simulink library "xrbsComm_r4"  (Simulink 7.1)
PreLoadFcn:
  | warning('off','MATLAB:mex:deprecatedExtension');xlmeta;com.xilinx.sysgen.util.StrategyUtil.loadAllStrategyNames();
undefined symbols (not defined in the file or in its folder): calc_path_data, gcbh, mfcm_matrix_rom, oct2dec, xlBlockLoadCallback
libraries: xbsIndex_r4 x851, mfcm_block_lib_v1 x5, xrbsComm_r4 x1, mfcm_misc_lib_v1 x1
(part 3 of 8)

== system xrbsComm_r4/White Gaussian  Noise Generator/Box-Muller1/f/lfsr_29_2 ==
  note: 4-Bit Leap-Forward LFSR G(X) = X^29 + X^2 + 1
  reset : Inport  OutDataType=sfix(16)  OutScaling=2^0
  Concat : xbsIndex_r4/Concat  num_inputs=2  dbl_ovrd=off  block_type=concat
      settings: block_version=VER_STRING_GOES_HERE
  Concat1 : xbsIndex_r4/Concat  num_inputs=2  dbl_ovrd=off  block_type=concat
      settings: block_version=VER_STRING_GOES_HERE
  Concat2 : xbsIndex_r4/Concat  num_inputs=2  dbl_ovrd=off  block_type=concat
      settings: block_version=VER_STRING_GOES_HERE
  Logical{,1..3} (4 alike) : xbsIndex_r4/Logical  logical_function=XOR  inputs=2  en=off  latency=0  precision=User Defined  arith_type=Unsigned  n_bits=1  bin_pt=0  align_bp=on  dbl_ovrd=off  block_type=logical
      settings: xl_area=[0, 0, 0, 0, 0, 0, 0]  block_version=VER_STRING_GOES_HERE
  x : xbsIndex_r4/Register  init=init(1)  rst=on  en=off  dbl_ovrd=off  block_type=register
      settings: xl_area=[0, 0, 0, 0, 0, 0, 0]  block_version=VER_STRING_GOES_HERE
  x2 : xbsIndex_r4/Register  init=init(2)  rst=on  en=off  dbl_ovrd=off  block_type=register
      settings: xl_area=[0, 0, 0, 0, 0, 0, 0]  block_version=VER_STRING_GOES_HERE
  x3 : xbsIndex_r4/Register  init=init(3)  rst=on  en=off  dbl_ovrd=off  block_type=register
      settings: xl_area=[0, 0, 0, 0, 0, 0, 0]  block_version=VER_STRING_GOES_HERE
  x4 : xbsIndex_r4/Register  init=init(4)  rst=on  en=off  dbl_ovrd=off  block_type=register
      settings: xl_area=[0, 0, 0, 0, 0, 0, 0]  block_version=VER_STRING_GOES_HERE
  x5 : Subsystem  mask{init=init(5:4:29)}
  x6 : Subsystem  mask{init=init(6:4:26)}
  x7 : Subsystem  mask{init=init(7:4:27)}
  x8 : Subsystem  mask{init=init(8:4:28)}
  " " : Outport  OutDataType=sfix(16)  OutScaling=2^0
  wires:
  Logical/1 -> x5/1(" ")
  Logical1/1 -> x6/1(" ")
  Logical2/1 -> x7/1(" ")
  Logical3/1 -> x8/1(" ")
  x5/1(z-7) -> x/1, Logical3/2
  x6/1(z-6) -> x2/1, Logical/2
  x7/1(z-6) -> x3/1
  x8/1(z-6) -> x4/1
  x/1 -> Logical1/1, Concat/1
  x2/1 -> Concat/2, Logical2/1
  Concat/1 -> Concat2/1
  x3/1 -> Concat1/1, Logical3/1, Logical1/2
  x4/1 -> Concat1/2, Logical2/2, Logical/1
  Concat1/1 -> Concat2/2
  Concat2/1 -> " "/1
  reset/1 -> x8/2(reset), x7/2(reset), x6/2(reset), x5/2(reset), x/2, x2/2, x3/2, x4/2

== system xrbsComm_r4/White Gaussian  Noise Generator/Box-Muller1/f/lfsr_31_2 ==
  note: 4-Bit Leap-Forward LFSR G(X) = X^31 + X^3 + 1
  reset : Inport  OutDataType=sfix(16)  OutScaling=2^0
  Concat : xbsIndex_r4/Concat  num_inputs=2  dbl_ovrd=off  block_type=concat
      settings: block_version=VER_STRING_GOES_HERE
  Concat1 : xbsIndex_r4/Concat  num_inputs=2  dbl_ovrd=off  block_type=concat
      settings: block_version=VER_STRING_GOES_HERE
  Concat2 : xbsIndex_r4/Concat  num_inputs=2  dbl_ovrd=off  block_type=concat
      settings: block_version=VER_STRING_GOES_HERE
  Logical{,1..3} (4 alike) : xbsIndex_r4/Logical  logical_function=XOR  inputs=2  en=off  latency=0  precision=User Defined  arith_type=Unsigned  n_bits=1  bin_pt=0  align_bp=on  dbl_ovrd=off  block_type=logical
      settings: xl_area=[0, 0, 0, 0, 0, 0, 0]  block_version=VER_STRING_GOES_HERE
  x : xbsIndex_r4/Register  init=init(1)  rst=on  en=off  dbl_ovrd=off  block_type=register
      settings: xl_area=[0, 0, 0, 0, 0, 0, 0]  block_version=VER_STRING_GOES_HERE
  x2 : xbsIndex_r4/Register  init=init(2)  rst=on  en=off  dbl_ovrd=off  block_type=register
      settings: xl_area=[0, 0, 0, 0, 0, 0, 0]  block_version=VER_STRING_GOES_HERE
  x3 : xbsIndex_r4/Register  init=init(3)  rst=on  en=off  dbl_ovrd=off  block_type=register
      settings: xl_area=[0, 0, 0, 0, 0, 0, 0]  block_version=VER_STRING_GOES_HERE
  x4 : xbsIndex_r4/Register  init=init(4)  rst=on  en=off  dbl_ovrd=off  block_type=register
      settings: xl_area=[0, 0, 0, 0, 0, 0, 0]  block_version=VER_STRING_GOES_HERE
  x5 : Subsystem  mask{init=init(5:4:29)}
  x6 : Subsystem  mask{init=init(6:4:30)}
  x7 : Subsystem  mask{init=init(7:4:31)}
  x8 : Subsystem  mask{init=init(8:4:28)}
  " " : Outport  OutDataType=sfix(16)  OutScaling=2^0
  wires:
  Logical/1 -> x5/1(" ")
  Logical1/1 -> x6/1(" ")
  Logical2/1 -> x7/1(" ")
  Logical3/1 -> x8/1(" ")
  x5/1(z-7) -> Logical/1, x/1
  x6/1(z-7) -> Logical1/1, x2/1
  x7/1(z-7) -> x3/1, Logical2/1
  x8/1(z-6) -> x4/1
  x/1 -> Concat/1, Logical3/1
  x2/1 -> Concat/2, Logical/2
  Concat/1 -> Concat2/1
  x3/1 -> Concat1/1, Logical1/2
  x4/1 -> Logical2/2, Concat1/2, Logical3/2
  Concat1/1 -> Concat2/2
  Concat2/1 -> " "/1
  reset/1 -> x5/2(reset), x6/2(reset), x7/2(reset), x8/2(reset), x/2, x2/2, x3/2, x4/2

== system xrbsComm_r4/White Gaussian  Noise Generator/Box-Muller1/f/lfsr_41_2 ==
  note: 4-Bit Leap-Forward LFSR G(X) = X^41 + X^3 + 1
  reset : Inport  OutDataType=sfix(16)  OutScaling=2^0
  Concat : xbsIndex_r4/Concat  num_inputs=2  dbl_ovrd=off  block_type=concat
      settings: block_version=VER_STRING_GOES_HERE
  Concat1 : xbsIndex_r4/Concat  num_inputs=2  dbl_ovrd=off  block_type=concat
      settings: block_version=VER_STRING_GOES_HERE
  Concat2 : xbsIndex_r4/Concat  num_inputs=2  dbl_ovrd=off  block_type=concat
      settings: block_version=VER_STRING_GOES_HERE
  Logical{,1..3} (4 alike) : xbsIndex_r4/Logical  logical_function=XOR  inputs=2  en=off  latency=0  precision=User Defined  arith_type=Unsigned  n_bits=1  bin_pt=0  align_bp=on  dbl_ovrd=off  block_type=logical
      settings: xl_area=[0, 0, 0, 0, 0, 0, 0]  block_version=VER_STRING_GOES_HERE
  x : xbsIndex_r4/Register  init=init(1)  rst=on  en=off  dbl_ovrd=off  block_type=register
      settings: xl_area=[0, 0, 0, 0, 0, 0, 0]  block_version=VER_STRING_GOES_HERE
  x1 : Subsystem  mask{init=init(6:4:38)}
  x2 : xbsIndex_r4/Register  init=init(2)  rst=on  en=off  dbl_ovrd=off  block_type=register
      settings: xl_area=[0, 0, 0, 0, 0, 0, 0]  block_version=VER_STRING_GOES_HERE
  x3 : xbsIndex_r4/Register  init=init(3)  rst=on  en=off  dbl_ovrd=off  block_type=register
      settings: xl_area=[0, 0, 0, 0, 0, 0, 0]  block_version=VER_STRING_GOES_HERE
  x4 : xbsIndex_r4/Register  init=init(4)  rst=on  en=off  dbl_ovrd=off  block_type=register
      settings: xl_area=[0, 0, 0, 0, 0, 0, 0]  block_version=VER_STRING_GOES_HERE
  x5 : Subsystem  mask{init=init(5:4:41)}
  x6 : Subsystem  mask{init=init(7:4:39)}
  x7 : Subsystem  mask{init=init(8:4:40)}
  " " : Outport  OutDataType=sfix(16)  OutScaling=2^0
  wires:
  Logical/1 -> x5/1(" ")
  Logical1/1 -> x1/1(" ")
  Logical2/1 -> x6/1(" ")
  Logical3/1 -> x7/1(" ")
  x5/1(z-10) -> x/1, Logical2/2
  x1/1(z-9) -> x2/1, Logical3/2
  x6/1(z-9) -> x3/1, Logical/2
  x7/1(z-9) -> x4/1
  x/1 -> Logical1/1, Concat/1
  x2/1 -> Concat/2, Logical2/1
  Concat/1 -> Concat2/1
  x3/1 -> Concat1/1, Logical3/1
  x4/1 -> Concat1/2, Logical1/2, Logical/1
  Concat1/1 -> Concat2/2
  Concat2/1 -> " "/1
  reset/1 -> x5/2(reset), x1/2(reset), x6/2(reset), x7/2(reset), x/2, x2/2, x3/2, x4/2

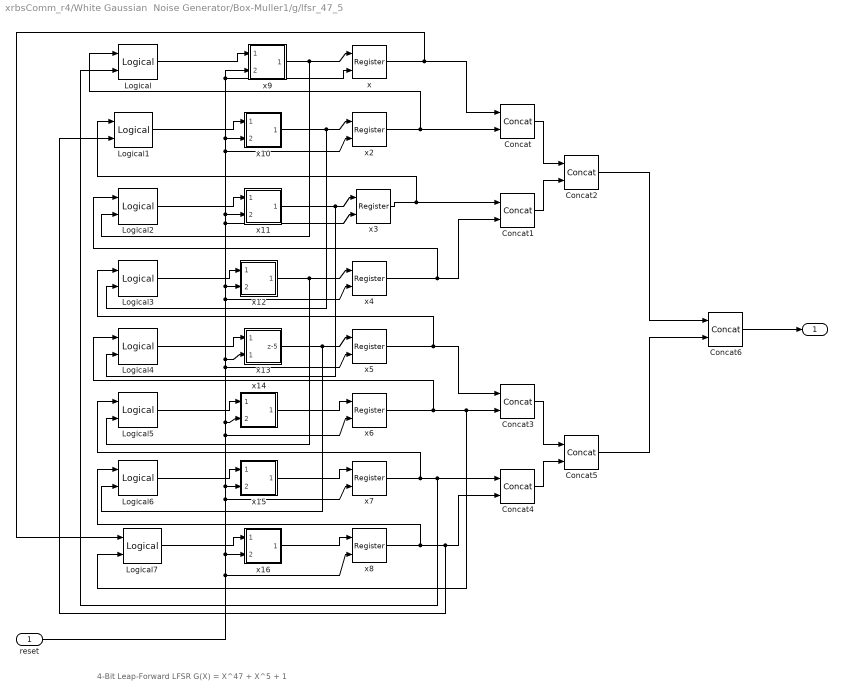
== system xrbsComm_r4/White Gaussian  Noise Generator/Box-Muller1/g/lfsr_47_5 ==
  note: 4-Bit Leap-Forward LFSR G(X) = X^47 + X^5 + 1
  reset : Inport  OutDataType=sfix(16)  OutScaling=2^0
  Concat{,1..6} (7 alike) : xbsIndex_r4/Concat  num_inputs=2  dbl_ovrd=off  block_type=concat
      settings: block_version=VER_STRING_GOES_HERE
  Logical{,1..7} (8 alike) : xbsIndex_r4/Logical  logical_function=XOR  inputs=2  en=off  latency=0  precision=User Defined  arith_type=Unsigned  n_bits=1  bin_pt=0  align_bp=on  dbl_ovrd=off  block_type=logical
      settings: xl_area=[0, 0, 0, 0, 0, 0, 0]  block_version=VER_STRING_GOES_HERE
  x : xbsIndex_r4/Register  init=init(1)  rst=on  en=off  dbl_ovrd=off  block_type=register
      settings: xl_area=[0, 0, 0, 0, 0, 0, 0]  block_version=VER_STRING_GOES_HERE
  x10 : Subsystem  mask{init=init(10:8:42)}
  x11 : Subsystem  mask{init=init(11:8:43)}
  x12 : Subsystem  mask{init=init(12:8:44)}
  x13 : Subsystem  mask{init=init(13:8:45)}
  x14 : Subsystem  mask{init=init(14:8:46)}
  x15 : Subsystem  mask{init=init(15:8:47)}
  x16 : Subsystem  mask{init=init(16:8:40)}
  x2 : xbsIndex_r4/Register  init=init(2)  rst=on  en=off  dbl_ovrd=off  block_type=register
      settings: xl_area=[0, 0, 0, 0, 0, 0, 0]  block_version=VER_STRING_GOES_HERE
  x3 : xbsIndex_r4/Register  init=init(3)  rst=on  en=off  dbl_ovrd=off  block_type=register
      settings: xl_area=[0, 0, 0, 0, 0, 0, 0]  block_version=VER_STRING_GOES_HERE
  x4 : xbsIndex_r4/Register  init=init(4)  rst=on  en=off  dbl_ovrd=off  block_type=register
      settings: xl_area=[0, 0, 0, 0, 0, 0, 0]  block_version=VER_STRING_GOES_HERE
  x5 : xbsIndex_r4/Register  init=init(5)  rst=on  en=off  dbl_ovrd=off  block_type=register
      settings: xl_area=[0, 0, 0, 0, 0, 0, 0]  block_version=VER_STRING_GOES_HERE
  x6 : xbsIndex_r4/Register  init=init(6)  rst=on  en=off  dbl_ovrd=off  block_type=register
      settings: xl_area=[0, 0, 0, 0, 0, 0, 0]  block_version=VER_STRING_GOES_HERE
  x7 : xbsIndex_r4/Register  init=init(7)  rst=on  en=off  dbl_ovrd=off  block_type=register
      settings: xl_area=[0, 0, 0, 0, 0, 0, 0]  block_version=VER_STRING_GOES_HERE
  x8 : xbsIndex_r4/Register  init=init(8)  rst=on  en=off  dbl_ovrd=off  block_type=register
      settings: xl_area=[0, 0, 0, 0, 0, 0, 0]  block_version=VER_STRING_GOES_HERE
  x9 : Subsystem  mask{init=init(9:8:41)}
  " " : Outport  OutDataType=sfix(16)  OutScaling=2^0
  wires:
  Logical/1 -> x9/1(" ")
  x9/1(z-5) -> x/1, Logical2/2
  x/1 -> Concat/1, Logical7/1
  x2/1 -> Concat/2, Logical/1
  Concat/1 -> Concat2/1
  x3/1 -> Concat1/1, Logical1/1
  x4/1 -> Concat1/2, Logical2/1
  Concat1/1 -> Concat2/2
  Logical1/1 -> x10/1("  ")
  x10/1(z-5) -> x2/1, Logical3/2
  Logical2/1 -> x11/1(" ")
  x11/1(z-5) -> x3/1, Logical4/2
  Logical3/1 -> x12/1(" ")
  x12/1(z-5) -> x4/1, Logical5/2
  Logical4/1 -> x13/1(" ")
  x13/1(z-5) -> x5/1, Logical6/2
  Logical5/1 -> x14/1(" ")
  x14/1(z-5) -> x6/1
  Logical6/1 -> x15/1(" ")
  x15/1(z-5) -> x7/1
  Logical7/1 -> x16/1(" ")
  x16/1(z-4) -> x8/1
  x6/1 -> Logical4/1, Concat3/2, Logical7/2
  Concat3/1 -> Concat5/1
  Concat4/1 -> Concat5/2
  x5/1 -> Concat3/1, Logical3/1
  x7/1 -> Concat4/1, Logical/2, Logical5/1
  x8/1 -> Concat4/2, Logical1/2, Logical6/1
  Concat2/1 -> Concat6/1
  Concat5/1 -> Concat6/2
  Concat6/1 -> " "/1
  reset/1 -> x9/2(reset), x/2, x10/2(reset), x2/2, x11/2(reset), x3/2, x12/2(reset), x4/2, x13/2(" 1"), x5/2, x14/2(reset), x6/2, x15/2(reset), x7/2, x16/2(reset), x8/2

== system xrbsComm_r4/White Gaussian  Noise Generator/Box-Muller2/fr1/iszero ==
  " " : Inport  OutDataType=sfix(16)  OutScaling=2^0
  "const " : xbsIndex_r4/Constant  arith_type=Unsigned  const=0  n_bits=4  bin_pt=0  explicit_period=off  period=1  equ=P=C  opselect=C  inp2=PCIN>>17  opr=+  inp1=P  carry=CIN  dbl_ovrd=off  block_type=constant
      settings: block_version=VER_STRING_GOES_HERE
  sel1 : xbsIndex_r4/Relational  mode=a=b  en=off  latency=1  dbl_ovrd=off  block_type=relational
      settings: xl_area=[0, 0, 0, 0, 0, 0, 0]  block_version=VER_STRING_GOES_HERE
  eq : Outport  OutDataType=sfix(16)  OutScaling=2^0
  wires:
  "const "/1 -> sel1/2
  " "/1 -> sel1/1
  sel1/1 -> eq/1

== system xrbsComm_r4/White Gaussian  Noise Generator/Box-Muller2/fr1/iszero1 ==
  " " : Inport  OutDataType=sfix(16)  OutScaling=2^0
  Constant1 : xbsIndex_r4/Constant  arith_type=Unsigned  const=0  n_bits=4  bin_pt=0  explicit_period=off  period=1  equ=P=C  opselect=C  inp2=PCIN>>17  opr=+  inp1=P  carry=CIN  dbl_ovrd=off  block_type=constant
      settings: block_version=VER_STRING_GOES_HERE
  sel2 : xbsIndex_r4/Relational  mode=a=b  en=off  latency=1  dbl_ovrd=off  block_type=relational
      settings: xl_area=[0, 0, 0, 0, 0, 0, 0]  block_version=VER_STRING_GOES_HERE
  eq : Outport  OutDataType=sfix(16)  OutScaling=2^0
  wires:
  Constant1/1 -> sel2/2
  " "/1 -> sel2/1
  sel2/1 -> eq/1

== system xrbsComm_r4/White Gaussian  Noise Generator/Box-Muller2/fr1/iszero2 ==
  " " : Inport  OutDataType=sfix(16)  OutScaling=2^0
  Constant3 : xbsIndex_r4/Constant  arith_type=Unsigned  const=0  n_bits=4  bin_pt=0  explicit_period=off  period=1  equ=P=C  opselect=C  inp2=PCIN>>17  opr=+  inp1=P  carry=CIN  dbl_ovrd=off  block_type=constant
      settings: block_version=VER_STRING_GOES_HERE
  sel3 : xbsIndex_r4/Relational  mode=a=b  en=off  latency=1  dbl_ovrd=off  block_type=relational
      settings: xl_area=[0, 0, 0, 0, 0, 0, 0]  block_version=VER_STRING_GOES_HERE
  eq : Outport  OutDataType=sfix(16)  OutScaling=2^0
  wires:
  Constant3/1 -> sel3/2
  " "/1 -> sel3/1
  sel3/1 -> eq/1

== system xrbsComm_r4/White Gaussian  Noise Generator/Box-Muller2/fr1/iszero3 ==
  " " : Inport  OutDataType=sfix(16)  OutScaling=2^0
  Constant : xbsIndex_r4/Constant  arith_type=Unsigned  const=0  n_bits=4  bin_pt=0  explicit_period=off  period=1  equ=P=C  opselect=C  inp2=PCIN>>17  opr=+  inp1=P  carry=CIN  dbl_ovrd=off  block_type=constant
      settings: block_version=VER_STRING_GOES_HERE
  sel4 : xbsIndex_r4/Relational  mode=a=b  en=off  latency=1  dbl_ovrd=off  block_type=relational
      settings: xl_area=[0, 0, 0, 0, 0, 0, 0]  block_version=VER_STRING_GOES_HERE
  eq : Outport  OutDataType=sfix(16)  OutScaling=2^0
  wires:
  Constant/1 -> sel4/2
  " "/1 -> sel4/1
  sel4/1 -> eq/1

== system xrbsComm_r4/White Gaussian  Noise Generator/Box-Muller2/fr1/lfsr_17_2 ==
  note: 4-Bit Leap-Forward LFSR G(X) = X^17 + X^3 + 1
  reset : Inport  OutDataType=sfix(16)  OutScaling=2^0
  Concat : xbsIndex_r4/Concat  num_inputs=2  dbl_ovrd=off  block_type=concat
      settings: block_version=VER_STRING_GOES_HERE
  Concat1 : xbsIndex_r4/Concat  num_inputs=2  dbl_ovrd=off  block_type=concat
      settings: block_version=VER_STRING_GOES_HERE
  Concat2 : xbsIndex_r4/Concat  num_inputs=2  dbl_ovrd=off  block_type=concat
      settings: block_version=VER_STRING_GOES_HERE
  Logical{,1..3} (4 alike) : xbsIndex_r4/Logical  logical_function=XOR  inputs=2  en=off  latency=0  precision=User Defined  arith_type=Unsigned  n_bits=1  bin_pt=0  align_bp=on  dbl_ovrd=off  block_type=logical
      settings: xl_area=[0, 0, 0, 0, 0, 0, 0]  block_version=VER_STRING_GOES_HERE
  x : xbsIndex_r4/Register  init=init(1)  rst=on  en=off  dbl_ovrd=off  block_type=register
      settings: xl_area=[0, 0, 0, 0, 0, 0, 0]  block_version=VER_STRING_GOES_HERE
  x1 : Subsystem  mask{init=init(7:4:15)}
  x2 : xbsIndex_r4/Register  init=init(2)  rst=on  en=off  dbl_ovrd=off  block_type=register
      settings: xl_area=[0, 0, 0, 0, 0, 0, 0]  block_version=VER_STRING_GOES_HERE
  x3 : xbsIndex_r4/Register  init=init(3)  rst=on  en=off  dbl_ovrd=off  block_type=register
      settings: xl_area=[0, 0, 0, 0, 0, 0, 0]  block_version=VER_STRING_GOES_HERE
  x4 : xbsIndex_r4/Register  init=init(4)  rst=on  en=off  dbl_ovrd=off  block_type=register
      settings: xl_area=[0, 0, 0, 0, 0, 0, 0]  block_version=VER_STRING_GOES_HERE
  x5 : Subsystem  mask{init=init(5:4:17)}
  x6 : Subsystem  mask{init=init(6:4:14)}
  x7 : Subsystem  mask{init=init(8:4:16)}
  " " : Outport  OutDataType=sfix(16)  OutScaling=2^0
  wires:
  Logical/1 -> x5/1(" ")
  Logical1/1 -> x6/1(" ")
  Logical2/1 -> x1/1(" ")
  Logical3/1 -> x7/1(" ")
  x5/1(z-4) -> x/1, Logical2/2
  x6/1(z-3) -> x2/1, Logical3/2
  x1/1(z-3) -> x3/1, Logical/2
  x7/1(z-3) -> x4/1
  x/1 -> Logical1/1, Concat/1
  x2/1 -> Concat/2, Logical2/1
  Concat/1 -> Concat2/1
  x3/1 -> Concat1/1, Logical3/1
  x4/1 -> Concat1/2, Logical1/2, Logical/1
  Concat1/1 -> Concat2/2
  Concat2/1 -> " "/1
  reset/1 -> x5/2(reset), x6/2(" reset"), x1/2(" reset"), x7/2(reset), x/2, x2/2, x3/2, x4/2

== system xrbsComm_r4/White Gaussian  Noise Generator/Box-Muller2/fr1/lfsr_25_2 ==
  note: 4-Bit Leap-Forward LFSR G(X) = X^25 + X^3 + 1
  " reset" : Inport  OutDataType=sfix(16)  OutScaling=2^0
  Concat : xbsIndex_r4/Concat  num_inputs=2  dbl_ovrd=off  block_type=concat
      settings: block_version=VER_STRING_GOES_HERE
  Concat1 : xbsIndex_r4/Concat  num_inputs=2  dbl_ovrd=off  block_type=concat
      settings: block_version=VER_STRING_GOES_HERE
  Concat2 : xbsIndex_r4/Concat  num_inputs=2  dbl_ovrd=off  block_type=concat
      settings: block_version=VER_STRING_GOES_HERE
  Logical{,1..3} (4 alike) : xbsIndex_r4/Logical  logical_function=XOR  inputs=2  en=off  latency=0  precision=User Defined  arith_type=Unsigned  n_bits=1  bin_pt=0  align_bp=on  dbl_ovrd=off  block_type=logical
      settings: xl_area=[0, 0, 0, 0, 0, 0, 0]  block_version=VER_STRING_GOES_HERE
  x : xbsIndex_r4/Register  init=init(1)  rst=on  en=off  dbl_ovrd=off  block_type=register
      settings: xl_area=[0, 0, 0, 0, 0, 0, 0]  block_version=VER_STRING_GOES_HERE
  x1 : Subsystem  mask{init=init(7:4:23)}
  x2 : xbsIndex_r4/Register  init=init(2)  rst=on  en=off  dbl_ovrd=off  block_type=register
      settings: xl_area=[0, 0, 0, 0, 0, 0, 0]  block_version=VER_STRING_GOES_HERE
  x3 : xbsIndex_r4/Register  init=init(3)  rst=on  en=off  dbl_ovrd=off  block_type=register
      settings: xl_area=[0, 0, 0, 0, 0, 0, 0]  block_version=VER_STRING_GOES_HERE
  x4 : xbsIndex_r4/Register  init=init(4)  rst=on  en=off  dbl_ovrd=off  block_type=register
      settings: xl_area=[0, 0, 0, 0, 0, 0, 0]  block_version=VER_STRING_GOES_HERE
  x5 : Subsystem  mask{init=init(5:4:25)}
  x6 : Subsystem  mask{init=init(6:4:22)}
  x7 : Subsystem  mask{init=init(8:4:24)}
  " " : Outport  OutDataType=sfix(16)  OutScaling=2^0
  wires:
  Concat2/1 -> " "/1
  Concat1/1 -> Concat2/2
  x4/1 -> Logical/1, Logical1/2, Concat1/2
  x3/1 -> Logical3/1, Concat1/1
  Concat/1 -> Concat2/1
  x/1 -> Concat/1, Logical1/1
  x7/1(z-5) -> x4/1
  x1/1(z-5) -> Logical/2, x3/1
  x6/1(z-5) -> Logical3/2, x2/1
  x5/1(z-6) -> Logical2/2, x/1
  Logical3/1 -> x7/1(" ")
  Logical2/1 -> x1/1(" ")
  Logical1/1 -> x6/1(" ")
  Logical/1 -> x5/1(" ")
  " reset"/1 -> x7/2(reset), x1/2(reset), x6/2(reset), x5/2(reset), x/2, x2/2, x3/2, x4/2
  x2/1 -> Concat/2, Logical2/1

== system xrbsComm_r4/White Gaussian  Noise Generator/Box-Muller2/fr1/lfsr_29_2 ==
  note: 4-Bit Leap-Forward LFSR G(X) = X^29 + X^2 + 1
  reset : Inport  OutDataType=sfix(16)  OutScaling=2^0
  Concat : xbsIndex_r4/Concat  num_inputs=2  dbl_ovrd=off  block_type=concat
      settings: block_version=VER_STRING_GOES_HERE
  Concat1 : xbsIndex_r4/Concat  num_inputs=2  dbl_ovrd=off  block_type=concat
      settings: block_version=VER_STRING_GOES_HERE
  Concat2 : xbsIndex_r4/Concat  num_inputs=2  dbl_ovrd=off  block_type=concat
      settings: block_version=VER_STRING_GOES_HERE
  Logical{,1..3} (4 alike) : xbsIndex_r4/Logical  logical_function=XOR  inputs=2  en=off  latency=0  precision=User Defined  arith_type=Unsigned  n_bits=1  bin_pt=0  align_bp=on  dbl_ovrd=off  block_type=logical
      settings: xl_area=[0, 0, 0, 0, 0, 0, 0]  block_version=VER_STRING_GOES_HERE
  x : xbsIndex_r4/Register  init=init(1)  rst=on  en=off  dbl_ovrd=off  block_type=register
      settings: xl_area=[0, 0, 0, 0, 0, 0, 0]  block_version=VER_STRING_GOES_HERE
  x2 : xbsIndex_r4/Register  init=init(2)  rst=on  en=off  dbl_ovrd=off  block_type=register
      settings: xl_area=[0, 0, 0, 0, 0, 0, 0]  block_version=VER_STRING_GOES_HERE
  x3 : xbsIndex_r4/Register  init=init(3)  rst=on  en=off  dbl_ovrd=off  block_type=register
      settings: xl_area=[0, 0, 0, 0, 0, 0, 0]  block_version=VER_STRING_GOES_HERE
  x4 : xbsIndex_r4/Register  init=init(4)  rst=on  en=off  dbl_ovrd=off  block_type=register
      settings: xl_area=[0, 0, 0, 0, 0, 0, 0]  block_version=VER_STRING_GOES_HERE
  x5 : Subsystem  mask{init=init(5:4:29)}
  x6 : Subsystem  mask{init=init(6:4:26)}
  x7 : Subsystem  mask{init=init(7:4:27)}
  x8 : Subsystem  mask{init=init(8:4:28)}
  " " : Outport  OutDataType=sfix(16)  OutScaling=2^0
  wires:
  Logical/1 -> x5/1(" ")
  Logical1/1 -> x6/1(" ")
  Logical2/1 -> x7/1(" ")
  Logical3/1 -> x8/1(" ")
  x5/1(z-7) -> x/1, Logical3/2
  x6/1(z-6) -> x2/1, Logical/2
  x7/1(z-6) -> x3/1
  x8/1(z-6) -> x4/1
  x/1 -> Logical1/1, Concat/1
  x2/1 -> Concat/2, Logical2/1
  Concat/1 -> Concat2/1
  x3/1 -> Concat1/1, Logical1/2, Logical3/1
  x4/1 -> Concat1/2, Logical2/2, Logical/1
  Concat1/1 -> Concat2/2
  Concat2/1 -> " "/1
  reset/1 -> x8/2(reset), x7/2(reset), x6/2(reset), x5/2(reset), x/2, x2/2, x3/2, x4/2

== system xrbsComm_r4/White Gaussian  Noise Generator/Box-Muller2/fr1/lfsr_31_2 ==
  note: 4-Bit Leap-Forward LFSR G(X) = X^31 + X^3 + 1
  reset : Inport  OutDataType=sfix(16)  OutScaling=2^0
  Concat : xbsIndex_r4/Concat  num_inputs=2  dbl_ovrd=off  block_type=concat
      settings: block_version=VER_STRING_GOES_HERE
  Concat1 : xbsIndex_r4/Concat  num_inputs=2  dbl_ovrd=off  block_type=concat
      settings: block_version=VER_STRING_GOES_HERE
  Concat2 : xbsIndex_r4/Concat  num_inputs=2  dbl_ovrd=off  block_type=concat
      settings: block_version=VER_STRING_GOES_HERE
  Logical{,1..3} (4 alike) : xbsIndex_r4/Logical  logical_function=XOR  inputs=2  en=off  latency=0  precision=User Defined  arith_type=Unsigned  n_bits=1  bin_pt=0  align_bp=on  dbl_ovrd=off  block_type=logical
      settings: xl_area=[0, 0, 0, 0, 0, 0, 0]  block_version=VER_STRING_GOES_HERE
  x : xbsIndex_r4/Register  init=init(1)  rst=on  en=off  dbl_ovrd=off  block_type=register
      settings: xl_area=[0, 0, 0, 0, 0, 0, 0]  block_version=VER_STRING_GOES_HERE
  x2 : xbsIndex_r4/Register  init=init(2)  rst=on  en=off  dbl_ovrd=off  block_type=register
      settings: xl_area=[0, 0, 0, 0, 0, 0, 0]  block_version=VER_STRING_GOES_HERE
  x3 : xbsIndex_r4/Register  init=init(3)  rst=on  en=off  dbl_ovrd=off  block_type=register
      settings: xl_area=[0, 0, 0, 0, 0, 0, 0]  block_version=VER_STRING_GOES_HERE
  x4 : xbsIndex_r4/Register  init=init(4)  rst=on  en=off  dbl_ovrd=off  block_type=register
      settings: xl_area=[0, 0, 0, 0, 0, 0, 0]  block_version=VER_STRING_GOES_HERE
  x5 : Subsystem  mask{init=init(5:4:29)}
  x6 : Subsystem  mask{init=init(6:4:30)}
  x7 : Subsystem  mask{init=init(7:4:31)}
  x8 : Subsystem  mask{init=init(8:4:28)}
  " " : Outport  OutDataType=sfix(16)  OutScaling=2^0
  wires:
  Logical/1 -> x5/1(" ")
  Logical1/1 -> x6/1(" ")
  Logical2/1 -> x7/1(" ")
  Logical3/1 -> x8/1(" ")
  x5/1(z-7) -> Logical/1, x/1
  x6/1(z-7) -> Logical1/1, x2/1
  x7/1(z-7) -> x3/1, Logical2/1
  x8/1(z-6) -> x4/1
  x/1 -> Concat/1, Logical3/1
  x2/1 -> Concat/2, Logical/2
  Concat/1 -> Concat2/1
  x3/1 -> Concat1/1, Logical1/2
  x4/1 -> Logical3/2, Concat1/2, Logical2/2
  Concat1/1 -> Concat2/2
  Concat2/1 -> " "/1
  reset/1 -> x7/2(reset), x5/2(reset), x6/2(reset), x8/2(reset), x/2, x2/2, x3/2, x4/2

== system xrbsComm_r4/White Gaussian  Noise Generator/Box-Muller2/fr1/lfsr_41_2 ==
  note: 4-Bit Leap-Forward LFSR G(X) = X^41 + X^3 + 1
  reset : Inport  OutDataType=sfix(16)  OutScaling=2^0
  Concat : xbsIndex_r4/Concat  num_inputs=2  dbl_ovrd=off  block_type=concat
      settings: block_version=VER_STRING_GOES_HERE
  Concat1 : xbsIndex_r4/Concat  num_inputs=2  dbl_ovrd=off  block_type=concat
      settings: block_version=VER_STRING_GOES_HERE
  Concat2 : xbsIndex_r4/Concat  num_inputs=2  dbl_ovrd=off  block_type=concat
      settings: block_version=VER_STRING_GOES_HERE
  Logical{,1..3} (4 alike) : xbsIndex_r4/Logical  logical_function=XOR  inputs=2  en=off  latency=0  precision=User Defined  arith_type=Unsigned  n_bits=1  bin_pt=0  align_bp=on  dbl_ovrd=off  block_type=logical
      settings: xl_area=[0, 0, 0, 0, 0, 0, 0]  block_version=VER_STRING_GOES_HERE
  x : xbsIndex_r4/Register  init=init(1)  rst=on  en=off  dbl_ovrd=off  block_type=register
      settings: xl_area=[0, 0, 0, 0, 0, 0, 0]  block_version=VER_STRING_GOES_HERE
  x1 : Subsystem  mask{init=init(6:4:38)}
  x2 : xbsIndex_r4/Register  init=init(2)  rst=on  en=off  dbl_ovrd=off  block_type=register
      settings: xl_area=[0, 0, 0, 0, 0, 0, 0]  block_version=VER_STRING_GOES_HERE
  x3 : xbsIndex_r4/Register  init=init(3)  rst=on  en=off  dbl_ovrd=off  block_type=register
      settings: xl_area=[0, 0, 0, 0, 0, 0, 0]  block_version=VER_STRING_GOES_HERE
  x4 : xbsIndex_r4/Register  init=init(4)  rst=on  en=off  dbl_ovrd=off  block_type=register
      settings: xl_area=[0, 0, 0, 0, 0, 0, 0]  block_version=VER_STRING_GOES_HERE
  x5 : Subsystem  mask{init=init(5:4:41)}
  x6 : Subsystem  mask{init=init(7:4:39)}
  x7 : Subsystem  mask{init=init(8:4:40)}
  " " : Outport  OutDataType=sfix(16)  OutScaling=2^0
  wires:
  Logical/1 -> x5/1(" ")
  Logical1/1 -> x1/1(" ")
  Logical2/1 -> x6/1(" ")
  Logical3/1 -> x7/1(" ")
  x5/1(z-10) -> x/1, Logical2/2
  x1/1(z-9) -> x2/1, Logical3/2
  x6/1(z-9) -> x3/1, Logical/2
  x7/1(z-9) -> x4/1
  x/1 -> Logical1/1, Concat/1
  x2/1 -> Concat/2, Logical2/1
  Concat/1 -> Concat2/1
  x3/1 -> Concat1/1, Logical3/1
  x4/1 -> Concat1/2, Logical1/2, Logical/1
  Concat1/1 -> Concat2/2
  Concat2/1 -> " "/1
  reset/1 -> x5/2(reset), x1/2(reset), x6/2(reset), x7/2(reset), x/2, x2/2, x3/2, x4/2

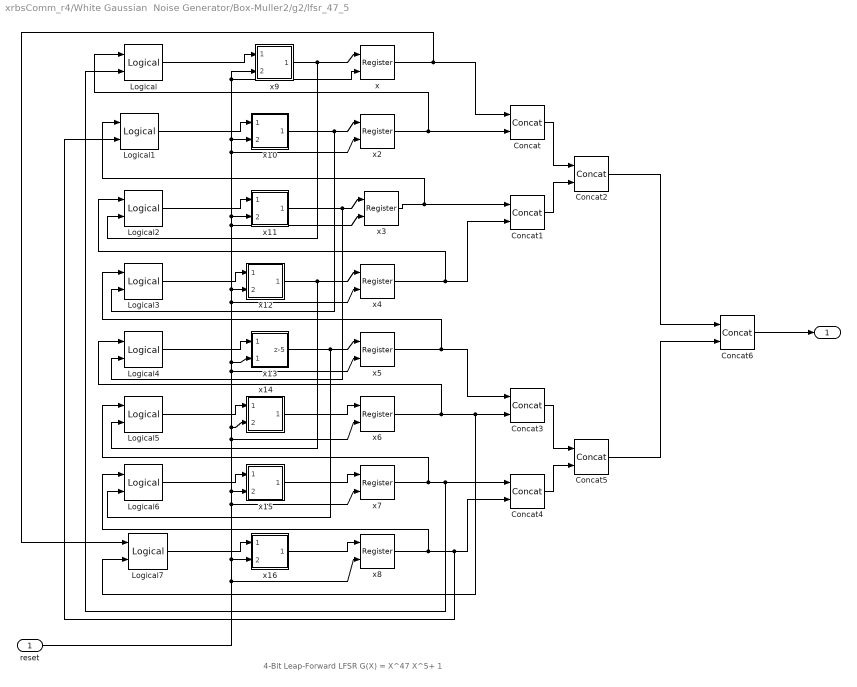
== system xrbsComm_r4/White Gaussian  Noise Generator/Box-Muller2/g2/lfsr_47_5 ==
  note: 4-Bit Leap-Forward LFSR G(X) = X^47 X^5+ 1
  reset : Inport  OutDataType=sfix(16)  OutScaling=2^0
  Concat{,1..6} (7 alike) : xbsIndex_r4/Concat  num_inputs=2  dbl_ovrd=off  block_type=concat
      settings: block_version=VER_STRING_GOES_HERE
  Logical{,1..7} (8 alike) : xbsIndex_r4/Logical  logical_function=XOR  inputs=2  en=off  latency=0  precision=User Defined  arith_type=Unsigned  n_bits=1  bin_pt=0  align_bp=on  dbl_ovrd=off  block_type=logical
      settings: xl_area=[0, 0, 0, 0, 0, 0, 0]  block_version=VER_STRING_GOES_HERE
  x : xbsIndex_r4/Register  init=init(1)  rst=on  en=off  dbl_ovrd=off  block_type=register
      settings: xl_area=[0, 0, 0, 0, 0, 0, 0]  block_version=VER_STRING_GOES_HERE
  x10 : Subsystem  mask{init=init(10:8:42)}
  x11 : Subsystem  mask{init=init(11:8:43)}
  x12 : Subsystem  mask{init=init(12:8:44)}
  x13 : Subsystem  mask{init=init(13:8:45)}
  x14 : Subsystem  mask{init=init(14:8:46)}
  x15 : Subsystem  mask{init=init(15:8:47)}
  x16 : Subsystem  mask{init=init(16:8:40)}
  x2 : xbsIndex_r4/Register  init=init(2)  rst=on  en=off  dbl_ovrd=off  block_type=register
      settings: xl_area=[0, 0, 0, 0, 0, 0, 0]  block_version=VER_STRING_GOES_HERE
  x3 : xbsIndex_r4/Register  init=init(3)  rst=on  en=off  dbl_ovrd=off  block_type=register
      settings: xl_area=[0, 0, 0, 0, 0, 0, 0]  block_version=VER_STRING_GOES_HERE
  x4 : xbsIndex_r4/Register  init=init(4)  rst=on  en=off  dbl_ovrd=off  block_type=register
      settings: xl_area=[0, 0, 0, 0, 0, 0, 0]  block_version=VER_STRING_GOES_HERE
  x5 : xbsIndex_r4/Register  init=init(5)  rst=on  en=off  dbl_ovrd=off  block_type=register
      settings: xl_area=[0, 0, 0, 0, 0, 0, 0]  block_version=VER_STRING_GOES_HERE
  x6 : xbsIndex_r4/Register  init=init(6)  rst=on  en=off  dbl_ovrd=off  block_type=register
      settings: xl_area=[0, 0, 0, 0, 0, 0, 0]  block_version=VER_STRING_GOES_HERE
  x7 : xbsIndex_r4/Register  init=init(7)  rst=on  en=off  dbl_ovrd=off  block_type=register
      settings: xl_area=[0, 0, 0, 0, 0, 0, 0]  block_version=VER_STRING_GOES_HERE
  x8 : xbsIndex_r4/Register  init=init(8)  rst=on  en=off  dbl_ovrd=off  block_type=register
      settings: xl_area=[0, 0, 0, 0, 0, 0, 0]  block_version=VER_STRING_GOES_HERE
  x9 : Subsystem  mask{init=init(9:8:41)}
  " " : Outport  OutDataType=sfix(16)  OutScaling=2^0
  wires:
  Logical/1 -> x9/1(" ")
  x9/1(z-5) -> x/1, Logical2/2
  x/1 -> Concat/1, Logical7/1
  x2/1 -> Concat/2, Logical/1
  Concat/1 -> Concat2/1
  x3/1 -> Concat1/1, Logical1/1
  x4/1 -> Concat1/2, Logical2/1
  Concat1/1 -> Concat2/2
  Logical1/1 -> x10/1("  ")
  x10/1(z-5) -> x2/1, Logical3/2
  Logical2/1 -> x11/1(" ")
  x11/1(z-5) -> x3/1, Logical4/2
  Logical3/1 -> x12/1(" ")
  x12/1(z-5) -> x4/1, Logical5/2
  Logical4/1 -> x13/1(" ")
  x13/1(z-5) -> x5/1, Logical6/2
  Logical5/1 -> x14/1(" ")
  x14/1(z-5) -> x6/1
  Logical6/1 -> x15/1(" ")
  x15/1(z-5) -> x7/1
  Logical7/1 -> x16/1(" ")
  x16/1(z-4) -> x8/1
  x6/1 -> Logical4/1, Concat3/2, Logical7/2
  Concat3/1 -> Concat5/1
  Concat4/1 -> Concat5/2
  x5/1 -> Concat3/1, Logical3/1
  x7/1 -> Concat4/1, Logical/2, Logical5/1
  x8/1 -> Concat4/2, Logical1/2, Logical6/1
  Concat2/1 -> Concat6/1
  Concat5/1 -> Concat6/2
  Concat6/1 -> " "/1
  reset/1 -> x9/2(reset), x/2, x10/2(reset), x2/2, x11/2(reset), x3/2, x12/2(reset), x4/2, x13/2(" 1"), x5/2, x14/2(reset), x6/2, x15/2(reset), x7/2, x16/2(reset), x8/2

== system xrbsComm_r4/White Gaussian  Noise Generator/Box-Muller3/fr1/iszero ==
  " " : Inport  OutDataType=sfix(16)  OutScaling=2^0
  "const " : xbsIndex_r4/Constant  arith_type=Unsigned  const=0  n_bits=4  bin_pt=0  explicit_period=off  period=1  equ=P=C  opselect=C  inp2=PCIN>>17  opr=+  inp1=P  carry=CIN  dbl_ovrd=off  block_type=constant
      settings: block_version=VER_STRING_GOES_HERE
  sel1 : xbsIndex_r4/Relational  mode=a=b  en=off  latency=1  dbl_ovrd=off  block_type=relational
      settings: xl_area=[0, 0, 0, 0, 0, 0, 0]  block_version=VER_STRING_GOES_HERE
  eq : Outport  OutDataType=sfix(16)  OutScaling=2^0
  wires:
  "const "/1 -> sel1/2
  " "/1 -> sel1/1
  sel1/1 -> eq/1

== system xrbsComm_r4/White Gaussian  Noise Generator/Box-Muller3/fr1/iszero1 ==
  " " : Inport  OutDataType=sfix(16)  OutScaling=2^0
  Constant1 : xbsIndex_r4/Constant  arith_type=Unsigned  const=0  n_bits=4  bin_pt=0  explicit_period=off  period=1  equ=P=C  opselect=C  inp2=PCIN>>17  opr=+  inp1=P  carry=CIN  dbl_ovrd=off  block_type=constant
      settings: block_version=VER_STRING_GOES_HERE
  sel2 : xbsIndex_r4/Relational  mode=a=b  en=off  latency=1  dbl_ovrd=off  block_type=relational
      settings: xl_area=[0, 0, 0, 0, 0, 0, 0]  block_version=VER_STRING_GOES_HERE
  eq : Outport  OutDataType=sfix(16)  OutScaling=2^0
  wires:
  Constant1/1 -> sel2/2
  " "/1 -> sel2/1
  sel2/1 -> eq/1

== system xrbsComm_r4/White Gaussian  Noise Generator/Box-Muller3/fr1/iszero2 ==
  " " : Inport  OutDataType=sfix(16)  OutScaling=2^0
  Constant3 : xbsIndex_r4/Constant  arith_type=Unsigned  const=0  n_bits=4  bin_pt=0  explicit_period=off  period=1  equ=P=C  opselect=C  inp2=PCIN>>17  opr=+  inp1=P  carry=CIN  dbl_ovrd=off  block_type=constant
      settings: block_version=VER_STRING_GOES_HERE
  sel3 : xbsIndex_r4/Relational  mode=a=b  en=off  latency=1  dbl_ovrd=off  block_type=relational
      settings: xl_area=[0, 0, 0, 0, 0, 0, 0]  block_version=VER_STRING_GOES_HERE
  eq : Outport  OutDataType=sfix(16)  OutScaling=2^0
  wires:
  Constant3/1 -> sel3/2
  " "/1 -> sel3/1
  sel3/1 -> eq/1

== system xrbsComm_r4/White Gaussian  Noise Generator/Box-Muller3/fr1/iszero3 ==
  " " : Inport  OutDataType=sfix(16)  OutScaling=2^0
  Constant : xbsIndex_r4/Constant  arith_type=Unsigned  const=0  n_bits=4  bin_pt=0  explicit_period=off  period=1  equ=P=C  opselect=C  inp2=PCIN>>17  opr=+  inp1=P  carry=CIN  dbl_ovrd=off  block_type=constant
      settings: block_version=VER_STRING_GOES_HERE
  sel4 : xbsIndex_r4/Relational  mode=a=b  en=off  latency=1  dbl_ovrd=off  block_type=relational
      settings: xl_area=[0, 0, 0, 0, 0, 0, 0]  block_version=VER_STRING_GOES_HERE
  eq : Outport  OutDataType=sfix(16)  OutScaling=2^0
  wires:
  Constant/1 -> sel4/2
  " "/1 -> sel4/1
  sel4/1 -> eq/1

== system xrbsComm_r4/White Gaussian  Noise Generator/Box-Muller3/fr1/lfsr_17_2 ==
  note: 4-Bit Leap-Forward LFSR G(X) = X^17 + X^3 + 1
  reset : Inport  OutDataType=sfix(16)  OutScaling=2^0
  Concat : xbsIndex_r4/Concat  num_inputs=2  dbl_ovrd=off  block_type=concat
      settings: block_version=VER_STRING_GOES_HERE
  Concat1 : xbsIndex_r4/Concat  num_inputs=2  dbl_ovrd=off  block_type=concat
      settings: block_version=VER_STRING_GOES_HERE
  Concat2 : xbsIndex_r4/Concat  num_inputs=2  dbl_ovrd=off  block_type=concat
      settings: block_version=VER_STRING_GOES_HERE
  Logical{,1..3} (4 alike) : xbsIndex_r4/Logical  logical_function=XOR  inputs=2  en=off  latency=0  precision=User Defined  arith_type=Unsigned  n_bits=1  bin_pt=0  align_bp=on  dbl_ovrd=off  block_type=logical
      settings: xl_area=[0, 0, 0, 0, 0, 0, 0]  block_version=VER_STRING_GOES_HERE
  x : xbsIndex_r4/Register  init=init(1)  rst=on  en=off  dbl_ovrd=off  block_type=register
      settings: xl_area=[0, 0, 0, 0, 0, 0, 0]  block_version=VER_STRING_GOES_HERE
  x1 : Subsystem  mask{init=init(7:4:15)}
  x2 : xbsIndex_r4/Register  init=init(2)  rst=on  en=off  dbl_ovrd=off  block_type=register
      settings: xl_area=[0, 0, 0, 0, 0, 0, 0]  block_version=VER_STRING_GOES_HERE
  x3 : xbsIndex_r4/Register  init=init(3)  rst=on  en=off  dbl_ovrd=off  block_type=register
      settings: xl_area=[0, 0, 0, 0, 0, 0, 0]  block_version=VER_STRING_GOES_HERE
  x4 : xbsIndex_r4/Register  init=init(4)  rst=on  en=off  dbl_ovrd=off  block_type=register
      settings: xl_area=[0, 0, 0, 0, 0, 0, 0]  block_version=VER_STRING_GOES_HERE
  x5 : Subsystem  mask{init=init(5:4:17)}
  x6 : Subsystem  mask{init=init(6:4:14)}
  x7 : Subsystem  mask{init=init(8:4:16)}
  " " : Outport  OutDataType=sfix(16)  OutScaling=2^0
  wires:
  Logical/1 -> x5/1(" ")
  Logical1/1 -> x6/1(" ")
  Logical2/1 -> x1/1(" ")
  Logical3/1 -> x7/1(" ")
  x5/1(z-4) -> x/1, Logical2/2
  x6/1(z-3) -> x2/1, Logical3/2
  x1/1(z-3) -> x3/1, Logical/2
  x7/1(z-3) -> x4/1
  x/1 -> Logical1/1, Concat/1
  x2/1 -> Concat/2, Logical2/1
  Concat/1 -> Concat2/1
  x3/1 -> Concat1/1, Logical3/1
  x4/1 -> Concat1/2, Logical1/2, Logical/1
  Concat1/1 -> Concat2/2
  Concat2/1 -> " "/1
  reset/1 -> x5/2(reset), x6/2(" reset"), x1/2(" reset"), x7/2(reset), x/2, x2/2, x3/2, x4/2

== system xrbsComm_r4/White Gaussian  Noise Generator/Box-Muller3/fr1/lfsr_25_2 ==
  note: 4-Bit Leap-Forward LFSR G(X) = X^25 + X^3 + 1
  " reset" : Inport  OutDataType=sfix(16)  OutScaling=2^0
  Concat : xbsIndex_r4/Concat  num_inputs=2  dbl_ovrd=off  block_type=concat
      settings: block_version=VER_STRING_GOES_HERE
  Concat1 : xbsIndex_r4/Concat  num_inputs=2  dbl_ovrd=off  block_type=concat
      settings: block_version=VER_STRING_GOES_HERE
  Concat2 : xbsIndex_r4/Concat  num_inputs=2  dbl_ovrd=off  block_type=concat
      settings: block_version=VER_STRING_GOES_HERE
  Logical{,1..3} (4 alike) : xbsIndex_r4/Logical  logical_function=XOR  inputs=2  en=off  latency=0  precision=User Defined  arith_type=Unsigned  n_bits=1  bin_pt=0  align_bp=on  dbl_ovrd=off  block_type=logical
      settings: xl_area=[0, 0, 0, 0, 0, 0, 0]  block_version=VER_STRING_GOES_HERE
  x : xbsIndex_r4/Register  init=init(1)  rst=on  en=off  dbl_ovrd=off  block_type=register
      settings: xl_area=[0, 0, 0, 0, 0, 0, 0]  block_version=VER_STRING_GOES_HERE
  x1 : Subsystem  mask{init=init(7:4:23)}
  x2 : xbsIndex_r4/Register  init=init(2)  rst=on  en=off  dbl_ovrd=off  block_type=register
      settings: xl_area=[0, 0, 0, 0, 0, 0, 0]  block_version=VER_STRING_GOES_HERE
  x3 : xbsIndex_r4/Register  init=init(3)  rst=on  en=off  dbl_ovrd=off  block_type=register
      settings: xl_area=[0, 0, 0, 0, 0, 0, 0]  block_version=VER_STRING_GOES_HERE
  x4 : xbsIndex_r4/Register  init=init(4)  rst=on  en=off  dbl_ovrd=off  block_type=register
      settings: xl_area=[0, 0, 0, 0, 0, 0, 0]  block_version=VER_STRING_GOES_HERE
  x5 : Subsystem  mask{init=init(5:4:25)}
  x6 : Subsystem  mask{init=init(6:4:22)}
  x7 : Subsystem  mask{init=init(8:4:24)}
  " " : Outport  OutDataType=sfix(16)  OutScaling=2^0
  wires:
  Concat2/1 -> " "/1
  Concat1/1 -> Concat2/2
  x4/1 -> Logical/1, Logical1/2, Concat1/2
  x3/1 -> Logical3/1, Concat1/1
  Concat/1 -> Concat2/1
  x2/1 -> Logical2/1, Concat/2
  x/1 -> Concat/1, Logical1/1
  x7/1(z-5) -> x4/1
  x1/1(z-5) -> Logical/2, x3/1
  x6/1(z-5) -> Logical3/2, x2/1
  x5/1(z-6) -> Logical2/2, x/1
  Logical3/1 -> x7/1(" ")
  Logical2/1 -> x1/1(" ")
  Logical1/1 -> x6/1(" ")
  Logical/1 -> x5/1(" ")
  " reset"/1 -> x7/2(reset), x1/2(reset), x6/2(reset), x5/2(reset), x/2, x2/2, x3/2, x4/2

== system xrbsComm_r4/White Gaussian  Noise Generator/Box-Muller3/fr1/lfsr_29_2 ==
  note: 4-Bit Leap-Forward LFSR G(X) = X^29 + X^2 + 1
  reset : Inport  OutDataType=sfix(16)  OutScaling=2^0
  Concat : xbsIndex_r4/Concat  num_inputs=2  dbl_ovrd=off  block_type=concat
      settings: block_version=VER_STRING_GOES_HERE
  Concat1 : xbsIndex_r4/Concat  num_inputs=2  dbl_ovrd=off  block_type=concat
      settings: block_version=VER_STRING_GOES_HERE
  Concat2 : xbsIndex_r4/Concat  num_inputs=2  dbl_ovrd=off  block_type=concat
      settings: block_version=VER_STRING_GOES_HERE
  Logical{,1..3} (4 alike) : xbsIndex_r4/Logical  logical_function=XOR  inputs=2  en=off  latency=0  precision=User Defined  arith_type=Unsigned  n_bits=1  bin_pt=0  align_bp=on  dbl_ovrd=off  block_type=logical
      settings: xl_area=[0, 0, 0, 0, 0, 0, 0]  block_version=VER_STRING_GOES_HERE
  x : xbsIndex_r4/Register  init=init(1)  rst=on  en=off  dbl_ovrd=off  block_type=register
      settings: xl_area=[0, 0, 0, 0, 0, 0, 0]  block_version=VER_STRING_GOES_HERE
  x2 : xbsIndex_r4/Register  init=init(2)  rst=on  en=off  dbl_ovrd=off  block_type=register
      settings: xl_area=[0, 0, 0, 0, 0, 0, 0]  block_version=VER_STRING_GOES_HERE
  x3 : xbsIndex_r4/Register  init=init(3)  rst=on  en=off  dbl_ovrd=off  block_type=register
      settings: xl_area=[0, 0, 0, 0, 0, 0, 0]  block_version=VER_STRING_GOES_HERE
  x4 : xbsIndex_r4/Register  init=init(4)  rst=on  en=off  dbl_ovrd=off  block_type=register
      settings: xl_area=[0, 0, 0, 0, 0, 0, 0]  block_version=VER_STRING_GOES_HERE
  x5 : Subsystem  mask{init=init(5:4:29)}
  x6 : Subsystem  mask{init=init(6:4:26)}
  x7 : Subsystem  mask{init=init(7:4:27)}
  x8 : Subsystem  mask{init=init(8:4:28)}
  " " : Outport  OutDataType=sfix(16)  OutScaling=2^0
  wires:
  Logical/1 -> x5/1(" ")
  Logical1/1 -> x6/1(" ")
  Logical2/1 -> x7/1(" ")
  Logical3/1 -> x8/1(" ")
  x5/1(z-7) -> x/1, Logical3/2
  x6/1(z-6) -> x2/1, Logical/2
  x7/1(z-6) -> x3/1
  x8/1(z-6) -> x4/1
  x/1 -> Logical1/1, Concat/1
  x2/1 -> Concat/2, Logical2/1
  Concat/1 -> Concat2/1
  x3/1 -> Concat1/1, Logical1/2, Logical3/1
  x4/1 -> Concat1/2, Logical2/2, Logical/1
  Concat1/1 -> Concat2/2
  Concat2/1 -> " "/1
  reset/1 -> x8/2(reset), x7/2(reset), x6/2(reset), x5/2(reset), x/2, x2/2, x3/2, x4/2

== system xrbsComm_r4/White Gaussian  Noise Generator/Box-Muller3/fr1/lfsr_31_2 ==
  note: 4-Bit Leap-Forward LFSR G(X) = X^31 + X^3 + 1
  reset : Inport  OutDataType=sfix(16)  OutScaling=2^0
  Concat : xbsIndex_r4/Concat  num_inputs=2  dbl_ovrd=off  block_type=concat
      settings: block_version=VER_STRING_GOES_HERE
  Concat1 : xbsIndex_r4/Concat  num_inputs=2  dbl_ovrd=off  block_type=concat
      settings: block_version=VER_STRING_GOES_HERE
  Concat2 : xbsIndex_r4/Concat  num_inputs=2  dbl_ovrd=off  block_type=concat
      settings: block_version=VER_STRING_GOES_HERE
  Logical{,1..3} (4 alike) : xbsIndex_r4/Logical  logical_function=XOR  inputs=2  en=off  latency=0  precision=User Defined  arith_type=Unsigned  n_bits=1  bin_pt=0  align_bp=on  dbl_ovrd=off  block_type=logical
      settings: xl_area=[0, 0, 0, 0, 0, 0, 0]  block_version=VER_STRING_GOES_HERE
  x : xbsIndex_r4/Register  init=init(1)  rst=on  en=off  dbl_ovrd=off  block_type=register
      settings: xl_area=[0, 0, 0, 0, 0, 0, 0]  block_version=VER_STRING_GOES_HERE
  x2 : xbsIndex_r4/Register  init=init(2)  rst=on  en=off  dbl_ovrd=off  block_type=register
      settings: xl_area=[0, 0, 0, 0, 0, 0, 0]  block_version=VER_STRING_GOES_HERE
  x3 : xbsIndex_r4/Register  init=init(3)  rst=on  en=off  dbl_ovrd=off  block_type=register
      settings: xl_area=[0, 0, 0, 0, 0, 0, 0]  block_version=VER_STRING_GOES_HERE
  x4 : xbsIndex_r4/Register  init=init(4)  rst=on  en=off  dbl_ovrd=off  block_type=register
      settings: xl_area=[0, 0, 0, 0, 0, 0, 0]  block_version=VER_STRING_GOES_HERE
  x5 : Subsystem  mask{init=init(5:4:29)}
  x6 : Subsystem  mask{init=init(6:4:30)}
  x7 : Subsystem  mask{init=init(7:4:31)}
  x8 : Subsystem  mask{init=init(8:4:28)}
  " " : Outport  OutDataType=sfix(16)  OutScaling=2^0
  wires:
  Logical/1 -> x5/1(" ")
  Logical1/1 -> x6/1(" ")
  Logical2/1 -> x7/1(" ")
  Logical3/1 -> x8/1(" ")
  x5/1(z-7) -> Logical/1, x/1
  x6/1(z-7) -> Logical1/1, x2/1
  x7/1(z-7) -> x3/1, Logical2/1
  x8/1(z-6) -> x4/1
  x/1 -> Concat/1, Logical3/1
  x2/1 -> Concat/2, Logical/2
  Concat/1 -> Concat2/1
  x3/1 -> Concat1/1, Logical1/2
  x4/1 -> Logical2/2, Concat1/2, Logical3/2
  Concat1/1 -> Concat2/2
  Concat2/1 -> " "/1
  reset/1 -> x/2, x2/2, x3/2, x4/2, x5/2(reset), x6/2(reset), x7/2(reset), x8/2(reset)

== system xrbsComm_r4/White Gaussian  Noise Generator/Box-Muller3/fr1/lfsr_41_2 ==
  note: 4-Bit Leap-Forward LFSR G(X) = X^41 + X^3 + 1
  reset : Inport  OutDataType=sfix(16)  OutScaling=2^0
  Concat : xbsIndex_r4/Concat  num_inputs=2  dbl_ovrd=off  block_type=concat
      settings: block_version=VER_STRING_GOES_HERE
  Concat1 : xbsIndex_r4/Concat  num_inputs=2  dbl_ovrd=off  block_type=concat
      settings: block_version=VER_STRING_GOES_HERE
  Concat2 : xbsIndex_r4/Concat  num_inputs=2  dbl_ovrd=off  block_type=concat
      settings: block_version=VER_STRING_GOES_HERE
  Logical{,1..3} (4 alike) : xbsIndex_r4/Logical  logical_function=XOR  inputs=2  en=off  latency=0  precision=User Defined  arith_type=Unsigned  n_bits=1  bin_pt=0  align_bp=on  dbl_ovrd=off  block_type=logical
      settings: xl_area=[0, 0, 0, 0, 0, 0, 0]  block_version=VER_STRING_GOES_HERE
  x : xbsIndex_r4/Register  init=init(1)  rst=on  en=off  dbl_ovrd=off  block_type=register
      settings: xl_area=[0, 0, 0, 0, 0, 0, 0]  block_version=VER_STRING_GOES_HERE
  x1 : Subsystem  mask{init=init(6:4:38)}
  x2 : xbsIndex_r4/Register  init=init(2)  rst=on  en=off  dbl_ovrd=off  block_type=register
      settings: xl_area=[0, 0, 0, 0, 0, 0, 0]  block_version=VER_STRING_GOES_HERE
  x3 : xbsIndex_r4/Register  init=init(3)  rst=on  en=off  dbl_ovrd=off  block_type=register
      settings: xl_area=[0, 0, 0, 0, 0, 0, 0]  block_version=VER_STRING_GOES_HERE
  x4 : xbsIndex_r4/Register  init=init(4)  rst=on  en=off  dbl_ovrd=off  block_type=register
      settings: xl_area=[0, 0, 0, 0, 0, 0, 0]  block_version=VER_STRING_GOES_HERE
  x5 : Subsystem  mask{init=init(5:4:41)}
  x6 : Subsystem  mask{init=init(7:4:39)}
  x7 : Subsystem  mask{init=init(8:4:40)}
  " " : Outport  OutDataType=sfix(16)  OutScaling=2^0
  wires:
  Logical/1 -> x5/1(" ")
  Logical1/1 -> x1/1(" ")
  Logical2/1 -> x6/1(" ")
  Logical3/1 -> x7/1(" ")
  x5/1(z-10) -> x/1, Logical2/2
  x1/1(z-9) -> x2/1, Logical3/2
  x6/1(z-9) -> x3/1, Logical/2
  x7/1(z-9) -> x4/1
  x/1 -> Logical1/1, Concat/1
  x2/1 -> Concat/2, Logical2/1
  Concat/1 -> Concat2/1
  x3/1 -> Concat1/1, Logical3/1
  x4/1 -> Concat1/2, Logical/1, Logical1/2
  Concat1/1 -> Concat2/2
  Concat2/1 -> " "/1
  reset/1 -> x5/2(reset), x1/2(reset), x6/2(reset), x7/2(reset), x/2, x2/2, x3/2, x4/2

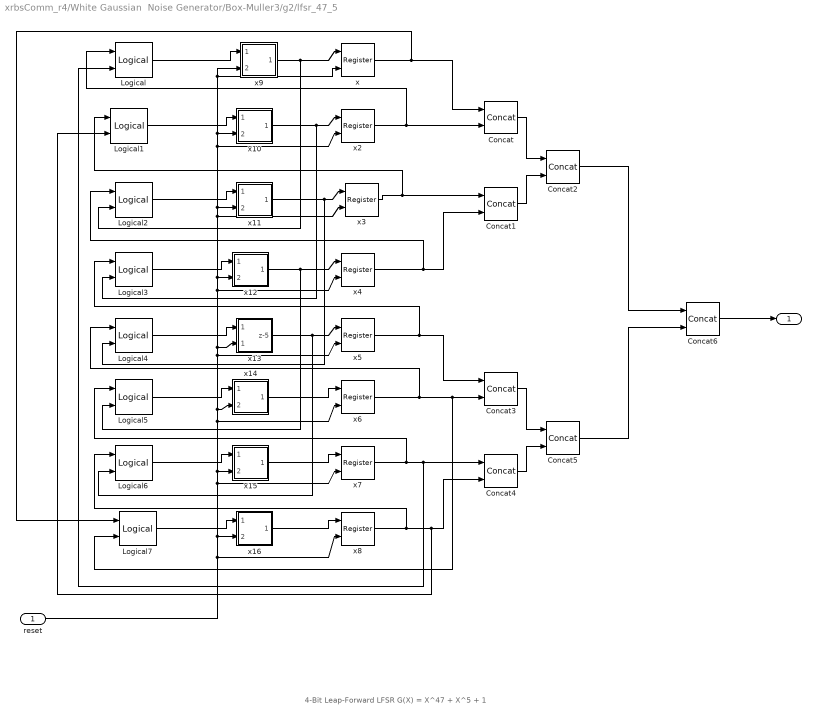
== system xrbsComm_r4/White Gaussian  Noise Generator/Box-Muller3/g2/lfsr_47_5 ==
  note: 4-Bit Leap-Forward LFSR G(X) = X^47 + X^5 + 1
  reset : Inport  OutDataType=sfix(16)  OutScaling=2^0
  Concat{,1..6} (7 alike) : xbsIndex_r4/Concat  num_inputs=2  dbl_ovrd=off  block_type=concat
      settings: block_version=VER_STRING_GOES_HERE
  Logical{,1..7} (8 alike) : xbsIndex_r4/Logical  logical_function=XOR  inputs=2  en=off  latency=0  precision=User Defined  arith_type=Unsigned  n_bits=1  bin_pt=0  align_bp=on  dbl_ovrd=off  block_type=logical
      settings: xl_area=[0, 0, 0, 0, 0, 0, 0]  block_version=VER_STRING_GOES_HERE
  x : xbsIndex_r4/Register  init=init(1)  rst=on  en=off  dbl_ovrd=off  block_type=register
      settings: xl_area=[0, 0, 0, 0, 0, 0, 0]  block_version=VER_STRING_GOES_HERE
  x10 : Subsystem  mask{init=init(10:8:42)}
  x11 : Subsystem  mask{init=init(11:8:43)}
  x12 : Subsystem  mask{init=init(12:8:44)}
  x13 : Subsystem  mask{init=init(13:8:45)}
  x14 : Subsystem  mask{init=init(14:8:46)}
  x15 : Subsystem  mask{init=init(15:8:47)}
  x16 : Subsystem  mask{init=init(16:8:40)}
  x2 : xbsIndex_r4/Register  init=init(2)  rst=on  en=off  dbl_ovrd=off  block_type=register
      settings: xl_area=[0, 0, 0, 0, 0, 0, 0]  block_version=VER_STRING_GOES_HERE
  x3 : xbsIndex_r4/Register  init=init(3)  rst=on  en=off  dbl_ovrd=off  block_type=register
      settings: xl_area=[0, 0, 0, 0, 0, 0, 0]  block_version=VER_STRING_GOES_HERE
  x4 : xbsIndex_r4/Register  init=init(4)  rst=on  en=off  dbl_ovrd=off  block_type=register
      settings: xl_area=[0, 0, 0, 0, 0, 0, 0]  block_version=VER_STRING_GOES_HERE
  x5 : xbsIndex_r4/Register  init=init(5)  rst=on  en=off  dbl_ovrd=off  block_type=register
      settings: xl_area=[0, 0, 0, 0, 0, 0, 0]  block_version=VER_STRING_GOES_HERE
  x6 : xbsIndex_r4/Register  init=init(6)  rst=on  en=off  dbl_ovrd=off  block_type=register
      settings: xl_area=[0, 0, 0, 0, 0, 0, 0]  block_version=VER_STRING_GOES_HERE
  x7 : xbsIndex_r4/Register  init=init(7)  rst=on  en=off  dbl_ovrd=off  block_type=register
      settings: xl_area=[0, 0, 0, 0, 0, 0, 0]  block_version=VER_STRING_GOES_HERE
  x8 : xbsIndex_r4/Register  init=init(8)  rst=on  en=off  dbl_ovrd=off  block_type=register
      settings: xl_area=[0, 0, 0, 0, 0, 0, 0]  block_version=VER_STRING_GOES_HERE
  x9 : Subsystem  mask{init=init(9:8:41)}
  " " : Outport  OutDataType=sfix(16)  OutScaling=2^0
  wires:
  Logical/1 -> x9/1(" ")
  x9/1(z-5) -> x/1, Logical2/2
  x/1 -> Concat/1, Logical7/1
  x2/1 -> Concat/2, Logical/1
  Concat/1 -> Concat2/1
  x3/1 -> Concat1/1, Logical1/1
  x4/1 -> Concat1/2, Logical2/1
  Concat1/1 -> Concat2/2
  Logical1/1 -> x10/1("  ")
  x10/1(z-5) -> x2/1, Logical3/2
  Logical2/1 -> x11/1(" ")
  x11/1(z-5) -> x3/1, Logical4/2
  Logical3/1 -> x12/1(" ")
  x12/1(z-5) -> x4/1, Logical5/2
  Logical4/1 -> x13/1(" ")
  x13/1(z-5) -> x5/1, Logical6/2
  Logical5/1 -> x14/1(" ")
  x14/1(z-5) -> x6/1
  Logical6/1 -> x15/1(" ")
  x15/1(z-5) -> x7/1
  Logical7/1 -> x16/1(" ")
  x16/1(z-4) -> x8/1
  x6/1 -> Logical4/1, Concat3/2, Logical7/2
  Concat3/1 -> Concat5/1
  Concat4/1 -> Concat5/2
  x5/1 -> Concat3/1, Logical3/1
  x7/1 -> Concat4/1, Logical/2, Logical5/1
  x8/1 -> Concat4/2, Logical1/2, Logical6/1
  Concat2/1 -> Concat6/1
  Concat5/1 -> Concat6/2
  Concat6/1 -> " "/1
  reset/1 -> x9/2(reset), x/2, x10/2(reset), x2/2, x11/2(reset), x3/2, x12/2(reset), x4/2, x13/2(" 1"), x5/2, x14/2(reset), x6/2, x15/2(reset), x7/2, x16/2(reset), x8/2

== system xrbsComm_r4/White Gaussian  Noise Generator/Box-Muller4/fr1/iszero ==
  " " : Inport  OutDataType=sfix(16)  OutScaling=2^0
  "const " : xbsIndex_r4/Constant  arith_type=Unsigned  const=0  n_bits=4  bin_pt=0  explicit_period=off  period=1  equ=P=C  opselect=C  inp2=PCIN>>17  opr=+  inp1=P  carry=CIN  dbl_ovrd=off  block_type=constant
      settings: block_version=VER_STRING_GOES_HERE
  sel1 : xbsIndex_r4/Relational  mode=a=b  en=off  latency=1  dbl_ovrd=off  block_type=relational
      settings: xl_area=[0, 0, 0, 0, 0, 0, 0]  block_version=VER_STRING_GOES_HERE
  eq : Outport  OutDataType=sfix(16)  OutScaling=2^0
  wires:
  "const "/1 -> sel1/2
  " "/1 -> sel1/1
  sel1/1 -> eq/1

== system xrbsComm_r4/White Gaussian  Noise Generator/Box-Muller4/fr1/iszero1 ==
  " " : Inport  OutDataType=sfix(16)  OutScaling=2^0
  Constant1 : xbsIndex_r4/Constant  arith_type=Unsigned  const=0  n_bits=4  bin_pt=0  explicit_period=off  period=1  equ=P=C  opselect=C  inp2=PCIN>>17  opr=+  inp1=P  carry=CIN  dbl_ovrd=off  block_type=constant
      settings: block_version=VER_STRING_GOES_HERE
  sel2 : xbsIndex_r4/Relational  mode=a=b  en=off  latency=1  dbl_ovrd=off  block_type=relational
      settings: xl_area=[0, 0, 0, 0, 0, 0, 0]  block_version=VER_STRING_GOES_HERE
  eq : Outport  OutDataType=sfix(16)  OutScaling=2^0
  wires:
  Constant1/1 -> sel2/2
  " "/1 -> sel2/1
  sel2/1 -> eq/1

== system xrbsComm_r4/White Gaussian  Noise Generator/Box-Muller4/fr1/iszero2 ==
  " " : Inport  OutDataType=sfix(16)  OutScaling=2^0
  Constant3 : xbsIndex_r4/Constant  arith_type=Unsigned  const=0  n_bits=4  bin_pt=0  explicit_period=off  period=1  equ=P=C  opselect=C  inp2=PCIN>>17  opr=+  inp1=P  carry=CIN  dbl_ovrd=off  block_type=constant
      settings: block_version=VER_STRING_GOES_HERE
  sel3 : xbsIndex_r4/Relational  mode=a=b  en=off  latency=1  dbl_ovrd=off  block_type=relational
      settings: xl_area=[0, 0, 0, 0, 0, 0, 0]  block_version=VER_STRING_GOES_HERE
  eq : Outport  OutDataType=sfix(16)  OutScaling=2^0
  wires:
  Constant3/1 -> sel3/2
  " "/1 -> sel3/1
  sel3/1 -> eq/1

== system xrbsComm_r4/White Gaussian  Noise Generator/Box-Muller4/fr1/iszero3 ==
  " " : Inport  OutDataType=sfix(16)  OutScaling=2^0
  Constant : xbsIndex_r4/Constant  arith_type=Unsigned  const=0  n_bits=4  bin_pt=0  explicit_period=off  period=1  equ=P=C  opselect=C  inp2=PCIN>>17  opr=+  inp1=P  carry=CIN  dbl_ovrd=off  block_type=constant
      settings: block_version=VER_STRING_GOES_HERE
  sel4 : xbsIndex_r4/Relational  mode=a=b  en=off  latency=1  dbl_ovrd=off  block_type=relational
      settings: xl_area=[0, 0, 0, 0, 0, 0, 0]  block_version=VER_STRING_GOES_HERE
  eq : Outport  OutDataType=sfix(16)  OutScaling=2^0
  wires:
  Constant/1 -> sel4/2
  " "/1 -> sel4/1
  sel4/1 -> eq/1
